simulink model "engine_R_2015b"  (R2015b)
settings: Solver=FixedStepDiscrete  SolverMode=SingleTasking  StartTime=0.0  StopTime=30.0  FixedStep=0.05  RelTol=1e-3
InitFcn:
  | loadvar
values from neighbouring files (symbols this model uses):
  x0 = [50, 50, 1.14275, 1.53787]    [loadvar.m]
settings Model: Creator=robin  LastModifiedBy=robin
settings DataIOCC: LimitDataPoints=off
settings DebuggingCC: AllowSymbolicDim=on  SFUnexpectedBacktrackingDiag=error  SFNoUnconditionalDefaultTransitionDiag=error
settings ModelReferenceCC: PropagateSignalLabelsOutOfModel=on
settings GRTTargetCC: TargetLangStandard=C99 (ISO)
settings ConfigComp: CovMetricSettings=dwe  CovHtmlReporting=off  CovSaveCumulativeToWorkspaceVar=off  CovSaveSingleToWorkspaceVar=off  CovModelRefEnable=Off  CovExternalEMLEnable=on

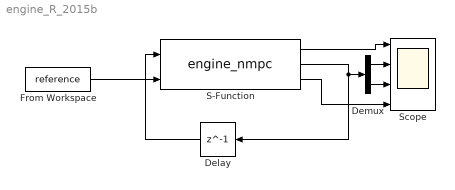
== system engine_R_2015b ==
  Delay : Delay  DelayLength=1  InitialCondition=x0
  Demux : Demux  Outputs=2
  From Workspace : FromWorkspace  VariableName=reference  SampleTime=0
  S-Function : S-Function  FunctionName=engine_nmpc  SFunctionDeploymentMode=off  EnableBusSupport=off
  Scope : Scope  NumInputPorts=4
  wires:
  S-Function/2 -> Demux/1, Delay/1
  Delay/1 -> S-Function/1
  S-Function/1 -> Scope/1
  S-Function/3 -> Scope/4
  Demux/1 -> Scope/2
  Demux/2 -> Scope/3
  From Workspace/1 -> S-Function/2
